simulink model "untitled"  (R2018a)
settings: Solver=VariableStepAuto  StartTime=0.0  StopTime=20  RelTol=1e-3
libraries: fuzblock x1
settings Model: Creator=xyoung  LastModifiedBy=80741

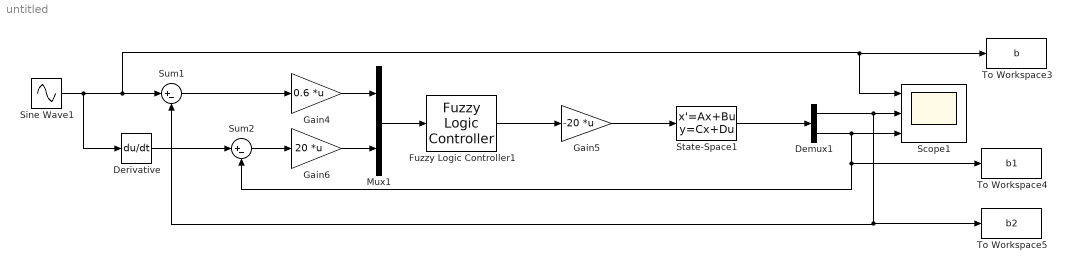
== system untitled ==
  Demux1 : Demux  Outputs=2
  Derivative : Derivative
  Fuzzy Logic Controller1 : fuzblock/Fuzzy Logic  Controller  FIS='Untitled.fis'  OutputSampleNumber=101  DataType=double  FuzzifiedInputs=off  RuleFiringStrengths=off  RuleOutputs=off  AggregatedOutputs=off  SimulateUsing=Interpreted execution  OutOfRangeInputValueMessage=warning  NoRuleFiredMessage=warning  EmptyOutputFuzzySetMessage=warning
  Gain4 : Gain  Gain=0.6  Multiplication=Matrix(K*u) (u vector)
  Gain5 : Gain  Gain=-20  Multiplication=Matrix(K*u) (u vector)
  Gain6 : Gain  Gain=20  Multiplication=Matrix(K*u) (u vector)
  Mux1 : Mux  Inputs=2
  Scope1 : Scope  NumInputPorts=3
  Sine Wave1 : Sin  Frequency=0.5  SampleTime=0
  State-Space1 : StateSpace  A=[0 0 0 1 0 0;0 0 0 0 1 0;0 0 0 0 0 1;0 1.0013 19.6166 0 0.0023 0.0078;0 -19.8594 -9.8083 0 -0.0451 -0.0039;0 -0.3004 -637.5397 0 -0.0007 -0.2537]  B=[0;0;0;0.1035;-0.0518;-0.0311]  C=[1 0 0 0 0 0;0 0 0 1 0 0]  D=[0;0]  InitialCondition=0
  Sum1 : Sum  Inputs=|+-
  Sum2 : Sum  Inputs=|+-
  To Workspace3 : ToWorkspace  VariableName=b  SaveFormat=Timeseries  SampleTime=-1
  To Workspace4 : ToWorkspace  VariableName=b1  SaveFormat=Timeseries  SampleTime=-1
  To Workspace5 : ToWorkspace  VariableName=b2  SaveFormat=Timeseries  SampleTime=-1
  wires:
  Demux1/1 -> To Workspace5/1, Sum1/2, Scope1/2
  Gain5/1 -> State-Space1/1
  Demux1/2 -> Scope1/3, Sum2/2, To Workspace4/1
  State-Space1/1 -> Demux1/1
  Gain6/1 -> Mux1/2
  Gain4/1 -> Mux1/1
  Fuzzy Logic Controller1/1 -> Gain5/1
  Sine Wave1/1 -> Derivative/1, To Workspace3/1, Scope1/1, Sum1/1
  Sum1/1 -> Gain4/1
  Mux1/1 -> Fuzzy Logic Controller1/1
  Sum2/1 -> Gain6/1
  Derivative/1 -> Sum2/1
